simulink model "Ref_LUT"  (R2015b)
settings: Solver=FixedStepDiscrete  SolverMode=SingleTasking  StartTime=0.0  StopTime=SimEnd+Ts2*NTaps*2  RelTol=1e-3
PreLoadFcn:
  | Param_fir
values from neighbouring files (symbols this model uses):
  NTaps = 128    [Param_fir.m]
  Numerator = firls(NTaps-1, [0 Fpass Fstop Fs/2]/(Fs/2), [1 1 0 0], [Wpass Wstop])    [Param_fir.m]
settings Model: Creator=bogilvie  LastModifiedBy=amatsumo
settings DataIOCC: SaveFormat=Array  SignalLoggingSaveFormat=ModelDataLogs  SaveOutput=off  SignalLogging=off  SaveTime=off
settings OptimizationCC: BlockReduction=off  ConditionallyExecuteInputs=off  DefaultParameterBehavior=Inlined  ExpressionDepthLimit=2147483647  InitFltsAndDblsToZero=on
settings DebuggingCC: AlgebraicLoopMsg=error  UnderspecifiedInitializationDetection=Classic  MergeDetectMultiDrivingBlocksExec=none  SignalResolutionControl=TryResolveAllWithWarning  SolverPrmCheckMsg=warning  SingleTaskRateTransMsg=error  IntegerOverflowMsg=none  ParameterOverflowMsg=warning  ParameterPrecisionLossMsg=none  FcnCallInpInsideContextMsg=UseLocalSettings  StateNameClashWarn=warning  IntegerSaturationMsg=none
settings HardwareCC: ProdBitPerPointer=32  ProdLargestAtomicFloat=None  ProdIntDivRoundTo=Undefined  ProdEndianess=Unspecified  ProdWordSize=32  ProdHWDeviceType=ASIC/FPGA->ASIC/FPGA  ProdEqTarget=off
settings SFSimCC: SFSimEcho=off
settings GRTTargetCC: GeneratePreprocessorConditionals=Disable all  CombineOutputUpdateFcns=off  GRTInterface=on
settings ConfigComp: CovModelRefEnable=Off  CovSFcnEnable=off

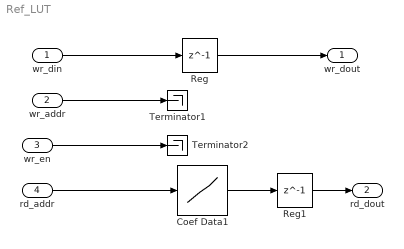
== system Ref_LUT ==
  wr_din : Inport  OutDataTypeStr=fixdt('sfix16_En15')  PortDimensions=1  SampleTime=[7.8125000000000002e-005,0]
  wr_addr : Inport  Port=2  OutDataTypeStr=fixdt('ufix7')  PortDimensions=1  SampleTime=[7.8125000000000002e-005,0]
  wr_en : Inport  Port=3  OutDataTypeStr=boolean  PortDimensions=1  SampleTime=[7.8125000000000002e-005,0]
  rd_addr : Inport  Port=4  OutDataTypeStr=fixdt('ufix7')  PortDimensions=1  SampleTime=[7.8125000000000002e-005,0]
  Coef Data1 : Lookup  InputValues=[0:NTaps-1]  Table=Numerator  LookUpMeth=Use Input Nearest  OutDataTypeStr=fixdt(1,16,15)
  Reg : Delay  DelayLength=1  InputProcessing=Inherited
  Reg1 : Delay  DelayLength=1  InputProcessing=Inherited
  Terminator1 : Terminator
  Terminator2 : Terminator
  wr_dout : Outport  OutDataTypeStr=fixdt('sfix16_En15')  PortDimensions=1  SampleTime=[7.8125000000000002e-005,0]
  rd_dout : Outport  Port=2  OutDataTypeStr=fixdt('sfix16_En15')  PortDimensions=1  SampleTime=[7.8125000000000002e-005,0]
  wires:
  Reg1/1 -> rd_dout/1
  Reg/1 -> wr_dout/1
  wr_en/1 -> Terminator2/1
  rd_addr/1 -> Coef Data1/1
  wr_din/1 -> Reg/1
  wr_addr/1 -> Terminator1/1
  Coef Data1/1 -> Reg1/1
